simulink model "task_1_sim"  (R2023a)
settings: Solver=VariableStepAuto  StartTime=0.0  StopTime=100  MaxStep=1e-4  RelTol=1e-4
undefined symbols (not defined in the file): A, B, Bw, C_Z, D_Z, K, x0
settings Model: Creator=user  LastModifiedBy=user

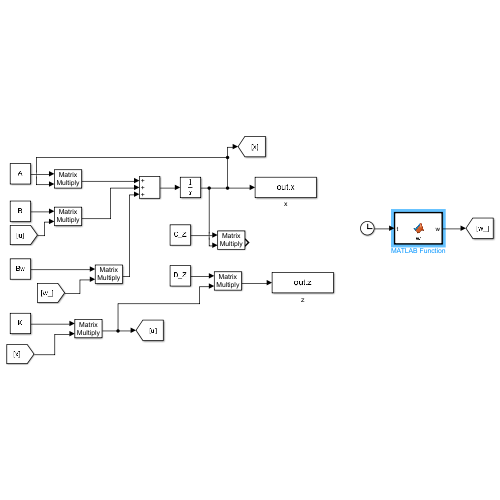
[thumbnail: Simulink's stored preview of the top-level diagram]
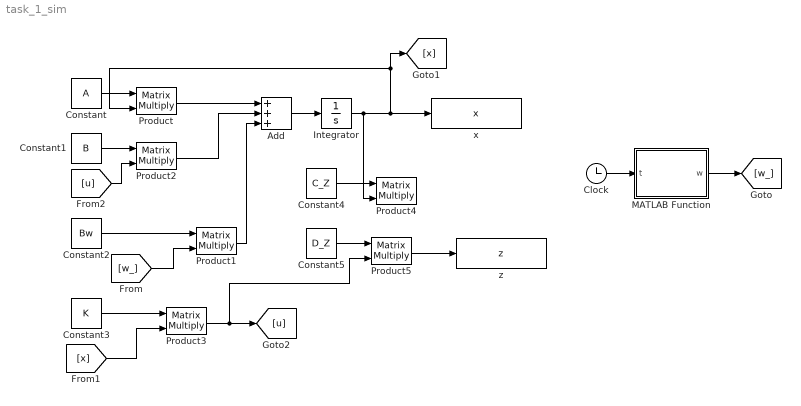
== system task_1_sim ==
  Add : Sum  Inputs=+++
  Clock : Clock
  Constant : Constant  Value=A  VectorParams1D=off
  Constant1 : Constant  Value=B  VectorParams1D=off
  Constant2 : Constant  Value=Bw  VectorParams1D=off
  Constant3 : Constant  Value=K  VectorParams1D=off
  Constant4 : Constant  Value=C_Z  VectorParams1D=off
  Constant5 : Constant  Value=D_Z  VectorParams1D=off
  Integrator : Integrator  InitialCondition=x0
  MATLAB Function : MATLAB Function  TreatAsAtomicUnit=on
  Product{,1..5} (6 alike) : Product  Multiplication=Matrix(*)
  x : ToWorkspace  VariableName=x  SaveFormat=Timeseries  SampleTime=-1
  z : ToWorkspace  VariableName=z  SaveFormat=Timeseries  SampleTime=-1
  wires:
  Clock/1 -> MATLAB Function/1(t)
  MATLAB Function/1(w) -> [w_]
  Integrator/1 -> Product4/2, Product/2, [x], x/1
  Constant/1 -> Product/1
  Add/1 -> Integrator/1
  Product/1 -> Add/1
  Constant3/1 -> Product3/1
  [x] -> Product3/2
  Product3/1 -> Product5/2, [u]
  Constant1/1 -> Product2/1
  [u] -> Product2/2
  Product2/1 -> Add/2
  Constant2/1 -> Product1/1
  [w_] -> Product1/2
  Product1/1 -> Add/3
  Constant4/1 -> Product4/1
  Constant5/1 -> Product5/1
  Product5/1 -> z/1

== matlab function task_1_sim/MATLAB Function ==
  data: t input; w output
function w = w(t)
    w = [1*sin(0.01*t);
         1*sin(0.05*t)];
    
end
